simulink model "Simulink-OFDM-16QAM"  (R2023b)
settings: Solver=ode45  StartTime=0.0  StopTime=0.01  RelTol=1e-3  EnableMultiTasking=on
undefined symbols (not defined in the file): doppler, Iter, Len, Max, Variance
libraries: dspobslib x6, commblkintrlv2 x6, dspindex x5, commsequence2 x5, commcnvcod2 x4, commchan3 x2, commcrc2 x2, commdigbbndam3 x2, dspxfrm3 x2, commseqgen3 x2, commutil2 x2, commrandsrc2 x1
settings Model: SimulationMode=accelerator  Creator=Administrator  LastModifiedBy=jackytu
settings SolverCC: AlgebraicLoopSolver=TrustRegion
settings DataIOCC: LimitDataPoints=on  SaveFormat=Array  ReturnWorkspaceOutputs=off
settings OptimizationCC: EfficientMapNaN2IntZero=off  LifeSpan=inf
settings DebuggingCC: SolverPrmCheckMsg=warning  UnconnectedInputMsg=warning  UnconnectedOutputMsg=warning  UnconnectedLineMsg=warning  SFUnexpectedBacktrackingDiag=warning  SFNoUnconditionalDefaultTransitionDiag=warning  SFExecutionAtInitializationDiag=none  ArithmeticOperatorsInVariantConditions=warning
settings HardwareCC: ProdBitPerPointer=32  ProdBitPerSizeT=32  ProdBitPerPtrDiffT=32  ProdLargestAtomicFloat=None  ProdIntDivRoundTo=Undefined  ProdEndianess=Unspecified  ProdWordSize=32  ProdHWDeviceType=32-bit Generic  TargetBitPerLong=64  TargetBitPerPointer=64  TargetBitPerSizeT=64  TargetBitPerPtrDiffT=64  TargetLongLongMode=on  TargetIntDivRoundTo=Zero  TargetEndianess=LittleEndian  TargetWordSize=64  TargetHWDeviceType=MATLAB Host  ProdEqTarget=off
settings ModelReferenceCC: PropagateSignalLabelsOutOfModel=off
settings SFSimCC: SimUseLocalCustomCode=off  CustomCodeUndefinedFunction=UseInterfaceOnly
settings RTWCC: RTWUseLocalCustomCode=off
settings CodeAppCC: MaxIdLength=128  StateflowObjectComments=on
settings GRTTargetCC: TargetLangStandard=C89/C90 (ANSI)  CombineOutputUpdateFcns=off  GRTInterface=on
settings ConfigComp: CovMetricSettings=dw  CovSaveCumulativeToWorkspaceVar=on  CovSaveSingleToWorkspaceVar=on  CovExternalEMLEnable=off  CovSFcnEnable=off

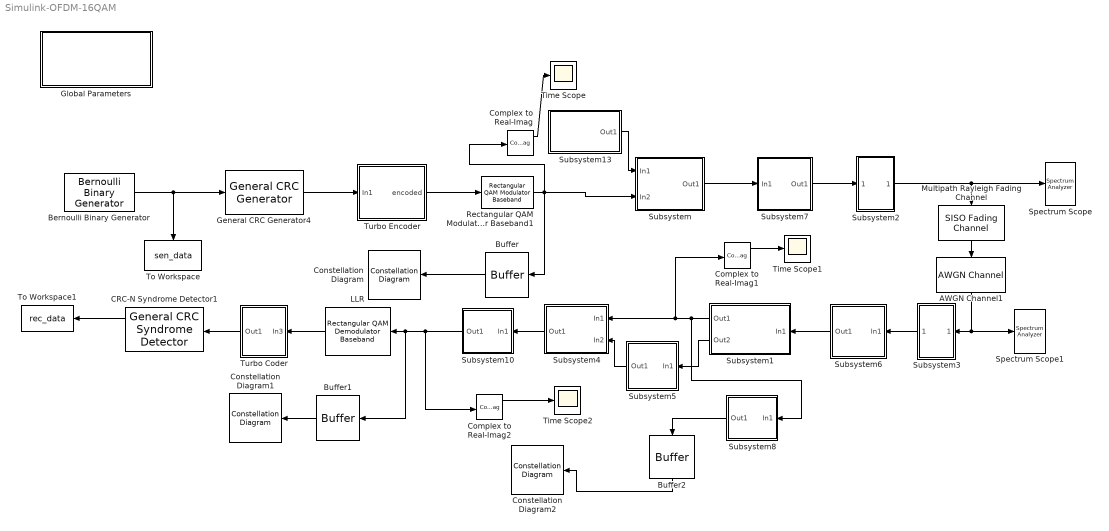
== system Simulink-OFDM-16QAM ==
  AWGN Channel1 : commchan3/AWGN Channel  LegacyMode=on  NoiseMethod="Signal to noise ratio  (SNR)"  noiseMode="Signal to noise ratio  (SNR)"  EbNo=10  EsNo=3  SNR=20  BitsPerSymbol=1  SignalPower=30/(5.5e5*11/15*2.4)*1.08  SamplesPerSymbol=1  SymbolPeriod=10e-5  VarianceSource=Parameter  Variance=1  RandomStream=Global stream  Seed=32965  SimulateUsing=Code generation
  Bernoulli Binary Generator : commrandsrc2/Bernoulli Binary Generator  P=0.5  seed=1000  Ts=10e-5/20  frameBased=on  sampPerFrame=20  orient=off  outDataType=boolean
  Buffer : Buffer  N=22*4
  Buffer1 : Buffer  N=22*4
  Buffer2 : Buffer  N=22*4
  CRC-N Syndrome Detector1 : commcrc2/General CRC Syndrome Detector  genPoly=[1 1 0 0 0 0 0 0 0 0 1 0 1 0 0 0 1 0 0 0 0 0 0 0 1]  iniStates=[0]  directMethod=off  reflectInputBytes=off  reflectChecksums=off  finalXOR=0  numChecksums=1
  Complex to Real-Imag : ComplexToRealImag
  Complex to Real-Imag1 : ComplexToRealImag
  Complex to Real-Imag2 : ComplexToRealImag
  Constellation Diagram : ConstellationDiagram  WindowPosition=[166.000000,185.000000,600.000000,600.000000,]  ScopeFrameLocation=window  DefaultConfigurationName=comm.scopes.ConstellationDiagramBlockCfg
  Constellation Diagram1 : ConstellationDiagram  WindowPosition=[945.000000,311.000000,600.000000,600.000000,]  ScopeFrameLocation=window  DefaultConfigurationName=comm.scopes.ConstellationDiagramBlockCfg
  Constellation Diagram2 : ConstellationDiagram  WindowPosition=[982.000000,81.000000,600.000000,600.000000,]  ScopeFrameLocation=window  DefaultConfigurationName=comm.scopes.ConstellationDiagramBlockCfg
  General CRC Generator4 : commcrc2/General CRC Generator  genPoly=[24,23,6,5,1,0]  iniStates=[0]  directMethod=off  reflectInputBytes=off  reflectChecksums=off  finalXOR=0  numChecksums=1
  Global Parameters : Subsystem  mask(Global Parameters){EbNodB=11, Len=44, Iter=5, Seed=54123}
      mask prompts: EbNodB "Eb/No in dB:"; Len "Block size:"; Iter "Number of iterations:"
      mask help: Load global parameters in MATLAB workspace.
      mask init:
      | turbo_code_punc_setup;
      mask Callback EbNodB: turbo_code_setup;
      mask Callback Len: turbo_code_setup
      mask Callback Iter: turbo_code_setup;
      mask Callback Seed: turbo_code_setup;
      mask Display: disp(['Eb/No ' num2str(EbNodB,'%3.1f') 'dB'  sprintf('\n') 'Block size   ' num2str(Len,'%7.0f')  sprintf('\n') 'Iterations   ' num2str(Iter,'%3.0f')   sprintf('\n') 'Seed   ' num2str(Seed,'%7.0f')])
  LLR : commdigbbndam3/Rectangular QAM Demodulator Baseband  M=16  OutType=Bit  DecType=Log-likelihood ratio  VarSource=Dialog  Variance=Variance  Dec=Gray  Mapping=[0:15]  PowType=Average Power  MinDist=2  AvgPow=0.5  PeakPow=1  Ph=0  outDtype1=double  outDtype2=double  derotateFactorWordLen=16  derotateFactorDataTypeStr=Inherit: Same word length as input  derotateFactorLastDataTypeStr=Inherit: Same word length as input  denormFactorWordLen=16  denormFactorDataTypeStr=Inherit: Same word length as input  denormFactorLastDataTypeStr=Inherit: Same word length as input  prodOutWordLen=32  prodOutOverflowMode=Wrap  prodOutRoundingMode=Floor  prodOutOvFlMode=off  prodOutOvFlModeLastStrValue=off  sumWordLen=32
  Multipath Rayleigh Fading Channel : commchan3/SISO Fading Channel  InheritSampleRate=on  SampleRate=1  PathDelays=[0 2e-6]  AveragePathGains=[0 -3]  NormalizePathGains=on  FadingDistribution=Rayleigh  KFactor=3  DirectPathDopplerShift=0  DirectPathInitialPhase=0  MaximumDopplerShift=400  DopplerSpectrum=doppler('Jakes')  RandomStream=mt19937ar with seed  Seed=73  PathGainsOutputPort=off  ChannelFilterDelayOutputPort=off  SimulateUsing=Interpreted execution  Visualization=Off  PathsForDopplerDisplay=1  SamplesToDisplay=25%
  Rectangular QAM Modulator Baseband1 : commdigbbndam3/Rectangular QAM Modulator Baseband  M=16  InType=Bit  Enc=Gray  Mapping=[0:15]  PowType=Average Power  MinDist=2  AvgPow=0.5  PeakPow=1  Ph=0  outDtype=double  outWordLen=16  outUDDataType=sfix(16)  outFracLenMode=Best precision  outFracLen=15  outDataTypeStr=double  outLastDataTypeStr=double
  Spectrum Scope : SpectrumAnalyzer  WindowPosition=[206.000000,125.000000,800.000000,500.000000,]  ScopeFrameLocation=window  Method=Welch  AveragingMethod=Running  YLimits=[-84.0138351,-3.23138917]  SelectedToolstripTab=spectrumAnalyzerToolstrip.spectrumTab  DefaultConfigurationName=spbscopes.SpectrumAnalyzerBlockCfg
  Spectrum Scope1 : SpectrumAnalyzer  WindowPosition=[742.000000,308.000000,800.000000,500.000000,]  ScopeFrameLocation=window  Method=Welch  AveragingMethod=Running  YLimits=[-78.17252741,-1.01212942]  SelectedToolstripTab=spectrumAnalyzerToolstrip.spectrumTab  DefaultConfigurationName=spbscopes.SpectrumAnalyzerBlockCfg
  Subsystem : Subsystem
      mask Display: disp('OFDM\nModulator')
  Subsystem1 : Subsystem
      mask Display: disp('OFDM\nDemodulator')
  Subsystem10 : Subsystem
      mask Display: disp('Remove\nZero')
  Subsystem13 : Subsystem
      mask Display: disp('Piolt Sequence')
  Subsystem2 : Subsystem
      mask Display: disp('P/S')
  Subsystem3 : Subsystem
      mask Display: disp('S/P')
  Subsystem4 : Subsystem
      mask Display: disp('Channel\nCompensation')
  Subsystem5 : Subsystem
      mask Display: disp('Channel\nEstimator')
  Subsystem6 : Subsystem
      mask Display: disp('Piolt\nSeparation')
  Subsystem7 : Subsystem
      mask Display: disp('Piolt\nInsertion')
  Subsystem8 : Subsystem
      mask Display: disp('Remove\nZero')
  Time Scope : Scope
  Time Scope1 : Scope
  Time Scope2 : Scope
  To Workspace : ToWorkspace  VariableName=sen_data  SampleTime=-1
  To Workspace1 : ToWorkspace  VariableName=rec_data  SampleTime=-1
  Turbo Coder : Subsystem
  Turbo Encoder : Subsystem
      mask Display: port_label('output',1,'Encoder');
  wires:
  Turbo Encoder/1(encoded) -> Rectangular QAM Modulator Baseband1/1
  Subsystem13/1(Out1) -> Subsystem/1(In1)
  Subsystem7/1(Out1) -> Subsystem2/1(In1)
  Rectangular QAM Modulator Baseband1/1 -> Complex to Real-Imag/1, Buffer/1, Subsystem/2(In2)
  Subsystem1/2(Out2) -> Subsystem5/1(In1)
  Subsystem5/1(Out1) -> Subsystem4/2(In2)
  Subsystem4/1(Out1) -> Subsystem10/1(In1)
  Subsystem3/1(Out1) -> Subsystem6/1(In1)
  Subsystem2/1(Out1) -> Multipath Rayleigh Fading Channel/1, Spectrum Scope/1
  AWGN Channel1/1 -> Spectrum Scope1/1, Subsystem3/1(In1)
  General CRC Generator4/1 -> Turbo Encoder/1(In1)
  Turbo Coder/1(Out1) -> CRC-N Syndrome Detector1/1
  Bernoulli Binary Generator/1 -> General CRC Generator4/1, To Workspace/1
  CRC-N Syndrome Detector1/1 -> To Workspace1/1
  Subsystem6/1(Out1) -> Subsystem1/1(In1)
  Subsystem/1(Out1) -> Subsystem7/1(In1)
  Multipath Rayleigh Fading Channel/1 -> AWGN Channel1/1
  LLR/1 -> Turbo Coder/1(In3)
  Complex to Real-Imag/1 -> Time Scope/1
  Buffer/1 -> Constellation Diagram/1
  Complex to Real-Imag1/1 -> Time Scope1/1
  Buffer1/1 -> Constellation Diagram1/1
  Subsystem1/1(Out1) -> Subsystem8/1(In1), Complex to Real-Imag1/1, Subsystem4/1(In1)
  Subsystem10/1(Out1) -> Complex to Real-Imag2/1, Buffer1/1, LLR/1
  Complex to Real-Imag2/1 -> Time Scope2/1
  Subsystem8/1(Out1) -> Buffer2/1
  Buffer2/1 -> Constellation Diagram2/1

== system Simulink-OFDM-16QAM/Global Parameters ==

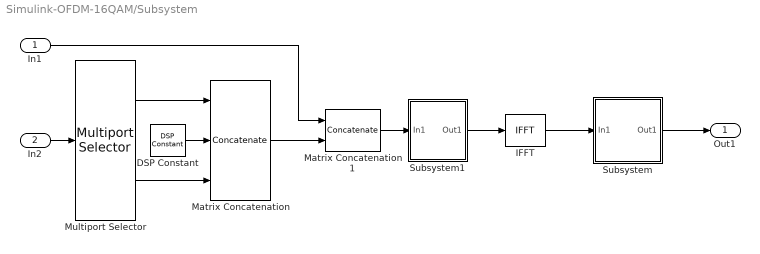
== system Simulink-OFDM-16QAM/Subsystem ==
  In1 : Inport
  In2 : Inport  Port=2
  DSP Constant : dspobslib/DSP Constant  Value=0  SampleMode=Discrete  discreteOutput=Frame-based  continuousOutput=Sample-based  sampTime=16e-5/2  framePeriod=10e-5  dataType=Inherit from 'Constant value'  isSigned=on  wordLen=16  udDataType=sfix(16)  fracBitsMode=Best precision  numFracBits=15  InterpretAs1D=off  Ts=16e-5/2  FramebasedOutput=on
  IFFT : dspxfrm3/IFFT  FFTImplementation=Auto  CompMethod=Table lookup  TableOpt=HYBRID  TableOptActive=Speed  BitRevOrder=off  cs_in=off  Normalize=on  InheritFFTLength=on  FFTLength=64  WrapInput=on  mode=Real  outSamplingMode=Frame based  roundingMode=Floor  overflowMode=off  firstCoeffDataTypeStr=Inherit: Same word length as input  firstCoeffLastDataTypeStr=Inherit: Same word length as input  outputMin=[]  outputMax=[]
  Matrix Concatenation : Concatenate  NumInputs=3  Mode=Multidimensional array
  Matrix Concatenation1 : Concatenate  Mode=Multidimensional array  ConcatenateDimension=2
  Multiport Selector : dspindex/Multiport Selector  rowsOrCols=Rows  idxCellArray={1:11,12:22}  idxErrMode=Clip Index
  Subsystem : Subsystem
      mask Display: disp('Add\nCyclic Prefix')
  Subsystem1 : Subsystem
      mask Display: disp('Zero Pad')
  Out1 : Outport
  wires:
  IFFT/1 -> Subsystem/1(In1)
  Multiport Selector/1 -> Matrix Concatenation/1
  Multiport Selector/2 -> Matrix Concatenation/3
  DSP Constant/1 -> Matrix Concatenation/2
  Subsystem1/1(Out1) -> IFFT/1
  Subsystem/1(Out1) -> Out1/1
  In2/1 -> Multiport Selector/1
  Matrix Concatenation1/1 -> Subsystem1/1(In1)
  Matrix Concatenation/1 -> Matrix Concatenation1/2
  In1/1 -> Matrix Concatenation1/1

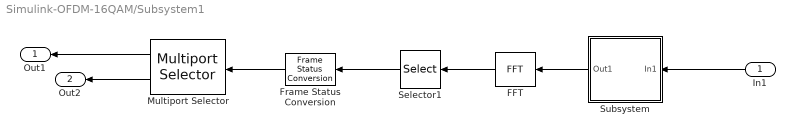
== system Simulink-OFDM-16QAM/Subsystem1 ==
  In1 : Inport
  FFT : dspxfrm3/FFT  FFTImplementation=Auto  CompMethod=Table lookup  TableOpt=HYBRID  TableOptActive=Speed  BitRevOrder=off  Normalize=on  InheritFFTLength=on  FFTLength=64  WrapInput=on  roundingMode=Floor  overflowMode=off  firstCoeffDataTypeStr=Inherit: Same word length as input  firstCoeffLastDataTypeStr=Inherit: Same word length as input  outputMin=[]  outputMax=[]
  Frame Status Conversion : dspobslib/Frame Status Conversion  growRefPort=off  outframe=Frame-based
  Multiport Selector : dspindex/Multiport Selector  rowsOrCols=Columns  idxCellArray={1,2}  idxErrMode=Clip Index
  Selector1 : Selector  NumberOfDimensions=2  InputPortWidth=64  IndexOptions=Index vector (dialog),Select all  Indices=[54:64,1:12],-1  OutputSizes=1
  Subsystem : Subsystem
      mask Display: disp('Remove\nCyclic Prefix')
  Out1 : Outport
  Out2 : Outport  Port=2
  wires:
  FFT/1 -> Selector1/1
  Selector1/1 -> Frame Status Conversion/1
  Subsystem/1(Out1) -> FFT/1
  Frame Status Conversion/1 -> Multiport Selector/1
  Multiport Selector/1 -> Out1/1
  Multiport Selector/2 -> Out2/1
  In1/1 -> Subsystem/1(In1)

== system Simulink-OFDM-16QAM/Subsystem10 ==
  In1 : Inport
  Selector2 : Selector  NumberOfDimensions=2  InputPortWidth=31  IndexOptions=Index vector (dialog),Select all  Indices=[1:11,13:23],-1  OutputSizes=1
  Out1 : Outport
  wires:
  Selector2/1 -> Out1/1
  In1/1 -> Selector2/1

== system Simulink-OFDM-16QAM/Subsystem13 ==
  PN Sequence Generator : commseqgen3/PN Sequence Generator  poly=[1 0 0 0 0 1 1]  ini_sta=[0 0 0 0 0 1]  outBitMaskSource=Dialog parameter  shift=0  outVarSiz=off  maxOutSizeMode=Dialog parameter  maxOutSize=[10 1]  Ts=10e-5/23  sampPerFrame=23  reset=off  bitPackedOutputs=off  outDataType=double  numPackedBits=8  bitPackDataSigned=off  bitPackedOutDType=double
  Unipolar to Bipolar Converter : commutil2/Unipolar to Bipolar Converter  M=2  polarity=Positive  dataType=Inherit via internal rule
  Out1 : Outport
  wires:
  PN Sequence Generator/1 -> Unipolar to Bipolar Converter/1
  Unipolar to Bipolar Converter/1 -> Out1/1

== system Simulink-OFDM-16QAM/Subsystem2 ==
  In1 : Inport
  Unbuffer3 : Unbuffer
  Out1 : Outport
  wires:
  In1/1 -> Unbuffer3/1
  Unbuffer3/1 -> Out1/1

== system Simulink-OFDM-16QAM/Subsystem3 ==
  In1 : Inport
  Buffer : Buffer  N=180
  Out1 : Outport
  wires:
  In1/1 -> Buffer/1
  Buffer/1 -> Out1/1

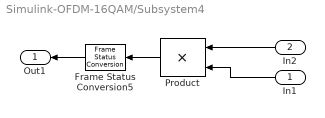
== system Simulink-OFDM-16QAM/Subsystem4 ==
  In1 : Inport
  In2 : Inport  Port=2
  Frame Status Conversion5 : dspobslib/Frame Status Conversion  growRefPort=off  outframe=Frame-based
  Product : Product  SaturateOnIntegerOverflow=on  OutDataTypeStr=Inherit: Same as first input
  Out1 : Outport
  wires:
  Product/1 -> Frame Status Conversion5/1
  Frame Status Conversion5/1 -> Out1/1
  In2/1 -> Product/1
  In1/1 -> Product/2

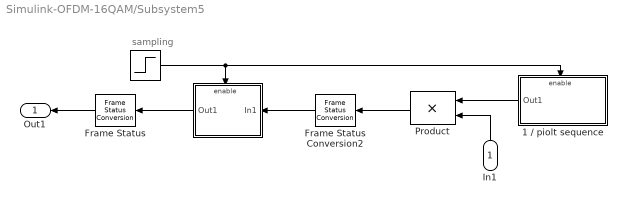
== system Simulink-OFDM-16QAM/Subsystem5 ==
  note: sampling
  In1 : Inport
  " " : Subsystem
      mask Display: disp('1\n----\nu');
  " " : Step  Time=10e-5  SampleTime=10e-5
  1 / piolt sequence : Subsystem  TreatAsAtomicUnit=on
      mask Display: disp('  1  \n-------\nPiolt');
  "Frame Status " : dspobslib/Frame Status Conversion  growRefPort=off  outframe=Frame-based
  Frame Status Conversion2 : dspobslib/Frame Status Conversion  growRefPort=off  outframe=Frame-based
  Product : Product  SaturateOnIntegerOverflow=on  OutDataTypeStr=Inherit: Same as first input
  Out1 : Outport
  wires:
  " "/1 -> 1 / piolt sequence/Enable, " "/Enable
  1 / piolt sequence/1(Out1) -> Product/1
  Product/1 -> Frame Status Conversion2/1
  Frame Status Conversion2/1 -> " "/1(In1)
  "Frame Status "/1 -> Out1/1
  In1/1 -> Product/2
  " "/1(Out1) -> "Frame Status "/1

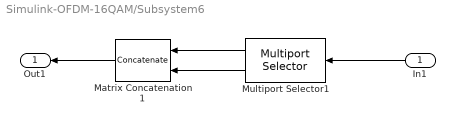
== system Simulink-OFDM-16QAM/Subsystem6 ==
  In1 : Inport
  Matrix Concatenation1 : Concatenate  Mode=Multidimensional array  ConcatenateDimension=2
  Multiport Selector1 : dspindex/Multiport Selector  rowsOrCols=Rows  idxCellArray={91:180,1:90}  idxErrMode=Clip Index
  Out1 : Outport
  wires:
  Multiport Selector1/2 -> Matrix Concatenation1/2
  Multiport Selector1/1 -> Matrix Concatenation1/1
  In1/1 -> Multiport Selector1/1
  Matrix Concatenation1/1 -> Out1/1

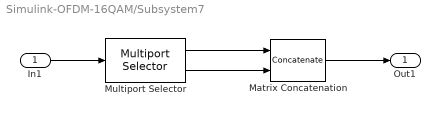
== system Simulink-OFDM-16QAM/Subsystem7 ==
  In1 : Inport
  Matrix Concatenation : Concatenate  Mode=Multidimensional array
  Multiport Selector : dspindex/Multiport Selector  rowsOrCols=Columns  idxCellArray={1,2}  idxErrMode=Clip Index
  Out1 : Outport
  wires:
  Multiport Selector/1 -> Matrix Concatenation/1
  Multiport Selector/2 -> Matrix Concatenation/2
  In1/1 -> Multiport Selector/1
  Matrix Concatenation/1 -> Out1/1

== system Simulink-OFDM-16QAM/Subsystem8 ==
  In1 : Inport
  Selector2 : Selector  NumberOfDimensions=2  InputPortWidth=31  IndexOptions=Index vector (dialog),Select all  Indices=[1:11,13:23],-1  OutputSizes=1
  Out1 : Outport
  wires:
  Selector2/1 -> Out1/1
  In1/1 -> Selector2/1

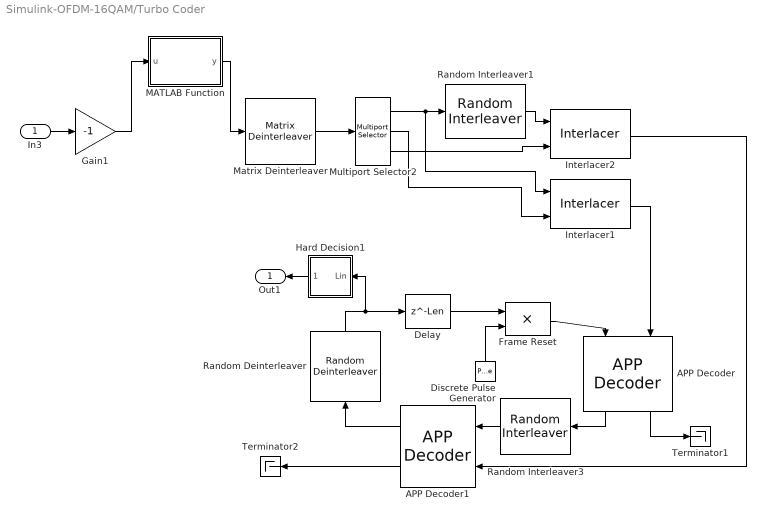
== system Simulink-OFDM-16QAM/Turbo Coder ==
  In3 : Inport
  APP Decoder : commcnvcod2/APP Decoder  trellis=trellis  termMethod=Truncated  algorithm=Max*  maxStarNumScaleBits=3  disableLcOut=off
  APP Decoder1 : commcnvcod2/APP Decoder  trellis=trellis  termMethod=Truncated  algorithm=Max*  maxStarNumScaleBits=3  disableLcOut=off
  Delay : Delay  DelayLength=Len  InitialCondition=0  InputProcessing=Columns as channels (frame based)
  Discrete Pulse Generator : DiscretePulseGenerator  Period=Iter  PulseWidth=Iter-1  PhaseDelay=1
  Frame Reset : Product  InputSameDT=on  SaturateOnIntegerOverflow=on  OutDataTypeStr=Inherit: Same as first input
  Gain1 : Gain  Gain=-1  SaturateOnIntegerOverflow=on  OutDataTypeStr=Inherit: Same as input  ParamDataTypeStr=Inherit: Same as input
  Hard Decision1 : Subsystem  mask(Hard Decision){}
      mask help: Likelihood to binary transformation.
  Interlacer1 : commsequence2/Interlacer
  Interlacer2 : commsequence2/Interlacer
  MATLAB Function : MATLAB Function  TreatAsAtomicUnit=on
  Matrix Deinterleaver : commblkintrlv2/Matrix Deinterleaver  Nrows=3  Ncols=44
  Multiport Selector2 : dspindex/Multiport Selector  rowsOrCols=Rows  idxCellArray={1:Len, Len+1:2*Len, 2*Len+1:3*Len}  idxErrMode=Clip Index
  Random Deinterleaver : commblkintrlv2/Random Deinterleaver  N=Len  seed=Seed
  Random Interleaver1 : commblkintrlv2/Random Interleaver  N=Len  seed=Seed
  Random Interleaver3 : commblkintrlv2/Random Interleaver  N=Len  seed=Seed
  Terminator1 : Terminator
  Terminator2 : Terminator
  Out1 : Outport
  wires:
  APP Decoder1/1 -> Random Deinterleaver/1
  APP Decoder/2 -> Terminator1/1
  APP Decoder1/2 -> Terminator2/1
  Random Deinterleaver/1 -> Delay/1, Hard Decision1/1(Lin)
  Random Interleaver3/1 -> APP Decoder1/1
  APP Decoder/1 -> Random Interleaver3/1
  Frame Reset/1 -> APP Decoder/1
  Delay/1 -> Frame Reset/1
  Discrete Pulse Generator/1 -> Frame Reset/2
  Hard Decision1/1(0/1) -> Out1/1
  Interlacer1/1 -> APP Decoder/2
  Interlacer2/1 -> APP Decoder1/2
  Multiport Selector2/1 -> Interlacer1/1, Random Interleaver1/1
  Multiport Selector2/2 -> Interlacer1/2
  Random Interleaver1/1 -> Interlacer2/1
  Multiport Selector2/3 -> Interlacer2/2
  Matrix Deinterleaver/1 -> Multiport Selector2/1
  In3/1 -> Gain1/1
  Gain1/1 -> MATLAB Function/1(u)
  MATLAB Function/1(y) -> Matrix Deinterleaver/1

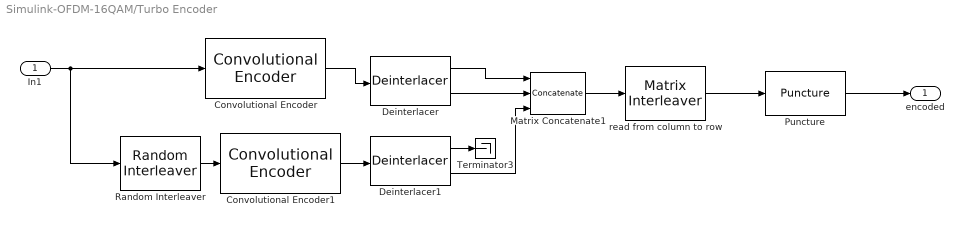
== system Simulink-OFDM-16QAM/Turbo Encoder ==
  In1 : Inport
  Convolutional Encoder : commcnvcod2/Convolutional Encoder  trellis=trellis  opMode=Continuous  DelayedResetAction=off  hasIniStPort=off  hasFinStPort=off  usePuncVector=off  punctureVector=[ 1 1 0 1 0 1]'  reset=Unused parameter value
  Convolutional Encoder1 : commcnvcod2/Convolutional Encoder  trellis=trellis  opMode=Truncated (reset every frame)  DelayedResetAction=off  hasIniStPort=off  hasFinStPort=off  usePuncVector=off  punctureVector=[ 1 1 0 1 0 1]'  reset=Unused parameter value
  Deinterlacer : commsequence2/Deinterlacer
  Deinterlacer1 : commsequence2/Deinterlacer
  Matrix Concatenate1 : Concatenate  NumInputs=3  Mode=Multidimensional array
  "Puncture " : commsequence2/Puncture  punctureVector=[1 1 0 1 0 1].'
  Random Interleaver : commblkintrlv2/Random Interleaver  N=Len  seed=Seed
  Terminator3 : Terminator
  read from column to row : commblkintrlv2/Matrix Interleaver  Nrows=3  Ncols=Len
  encoded : Outport
  wires:
  In1/1 -> Convolutional Encoder/1, Random Interleaver/1
  "Puncture "/1 -> encoded/1
  Random Interleaver/1 -> Convolutional Encoder1/1
  Convolutional Encoder/1 -> Deinterlacer/1
  Convolutional Encoder1/1 -> Deinterlacer1/1
  Deinterlacer1/1 -> Terminator3/1
  Deinterlacer/1 -> Matrix Concatenate1/1
  Deinterlacer1/2 -> Matrix Concatenate1/3
  read from column to row/1 -> "Puncture "/1
  Matrix Concatenate1/1 -> read from column to row/1
  Deinterlacer/2 -> Matrix Concatenate1/2

== system Simulink-OFDM-16QAM/Subsystem/Subsystem ==
  In1 : Inport
  Selector3 : Selector  NumberOfDimensions=2  InputPortWidth=64  IndexOptions=Index vector (dialog),Select all  Indices=[39:64,1:64],-1  OutputSizes=1
  Out1 : Outport
  wires:
  Selector3/1 -> Out1/1
  In1/1 -> Selector3/1

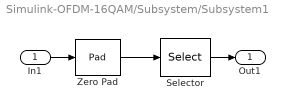
== system Simulink-OFDM-16QAM/Subsystem/Subsystem1 ==
  In1 : Inport
  Selector : Selector  NumberOfDimensions=2  InputPortWidth=64  IndexOptions=Index vector (dialog),Select all  Indices=[12:64,1:11],-1  OutputSizes=1
  Zero Pad : dspsigops/Pad  padAlong=Columns and rows  dimsToPad=1  valSrc=Specify via dialog  padVal=0  spec=Output size  padNumOutRowsSpecMethod=User-specified  numOutRows=64  padNumOutColsSpecMethod=User-specified  numOutCols=2  isVarDimsMode=off  padBeginning=0  padEnd=0  outSizeMode=User-specified  outSize=1  padSigAt=End  trunc_flag=None  roundingMode=Floor  overflowMode=off  truncOrWrapMode=Truncate  wrap_flag=None
  Out1 : Outport
  wires:
  Zero Pad/1 -> Selector/1
  In1/1 -> Zero Pad/1
  Selector/1 -> Out1/1

== system Simulink-OFDM-16QAM/Subsystem1/Subsystem ==
  In1 : Inport
  Selector4 : Selector  NumberOfDimensions=2  InputPortWidth=78  IndexOptions=Index vector (dialog),Select all  Indices=[27:90],-1  OutputSizes=1
  Out1 : Outport
  wires:
  Selector4/1 -> Out1/1
  In1/1 -> Selector4/1

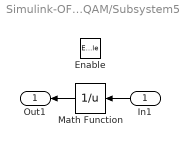
== system Simulink-OFDM-16QAM/Subsystem5/  ==
  In1 : Inport
  Enable : EnablePort
  Math Function : Math  Operator=reciprocal  SignedPower=on
  Out1 : Outport
  wires:
  In1/1 -> Math Function/1
  Math Function/1 -> Out1/1

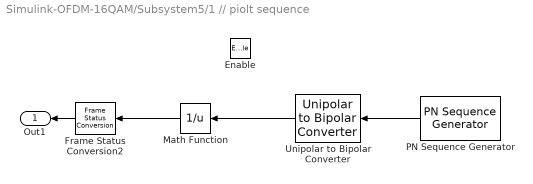
== system Simulink-OFDM-16QAM/Subsystem5/1 // piolt sequence ==
  Enable : EnablePort
  Frame Status Conversion2 : dspobslib/Frame Status Conversion  growRefPort=off  outframe=Frame-based
  Math Function : Math  Operator=reciprocal  SignedPower=on
  PN Sequence Generator : commseqgen3/PN Sequence Generator  poly=[1 0 0 0 0 1 1]  ini_sta=[0 0 0 0 0 1]  outBitMaskSource=Dialog parameter  shift=0  outVarSiz=off  maxOutSizeMode=Dialog parameter  maxOutSize=[10 1]  Ts=10e-5/23  sampPerFrame=23  reset=off  bitPackedOutputs=off  outDataType=double  numPackedBits=8  bitPackDataSigned=off  bitPackedOutDType=double
  Unipolar to Bipolar Converter : commutil2/Unipolar to Bipolar Converter  M=2  polarity=Positive  dataType=Inherit via internal rule
  Out1 : Outport
  wires:
  PN Sequence Generator/1 -> Unipolar to Bipolar Converter/1
  Frame Status Conversion2/1 -> Out1/1
  Math Function/1 -> Frame Status Conversion2/1
  Unipolar to Bipolar Converter/1 -> Math Function/1

== system Simulink-OFDM-16QAM/Turbo Coder/Hard Decision1 ==
  Lin : Inport
  Constant : Constant  Value=0
  Relational Operator : RelationalOperator
  0/1 : Outport
  wires:
  Constant/1 -> Relational Operator/2
  Lin/1 -> Relational Operator/1
  Relational Operator/1 -> 0/1/1

== matlab function Simulink-OFDM-16QAM/Turbo Coder/MATLAB Function ==
  data: u input; y output
function y = insertZeros(u)
    % This function inserts zeros into the input vector u according to
    % the specified pattern [1 1 0 1 0 1].
    
    % Define the pattern for inserting zeros
    pattern = [1; 1; 0; 1; 0; 1];
    patternLength = length(pattern);
    
    % Calculate how many times the pattern will be repeated
    numRepeats = length(u) / sum(pattern == 1);

    % Initialize output vector with zeros
    % The size of y will be the length of u plus the number of zeros to be inserted
    y = zeros(numRepeats * patternLength, 1);
    
    % Index for input vector
    uIdx = 1;
    
    % Insert input elements and zeros into the output vector
    for i = 1:numRepeats
        for pIdx = 1:patternLength
            if pattern(pIdx) == 1
                y((i-1)*patternLength + pIdx) = u(uIdx);
                uIdx = uIdx + 1;
            end
        end
    end
end
